simulink model "reactionWheel"  (R2019b)
settings: Solver=VariableStepAuto  StartTime=0.0  StopTime=10.0  RelTol=1e-3
model workspace (MAT data in the model file):
  Omega_max = 0.5
libraries: simulink x3, aerolibutil x1
settings Model: Creator=brice  LastModifiedBy=brice

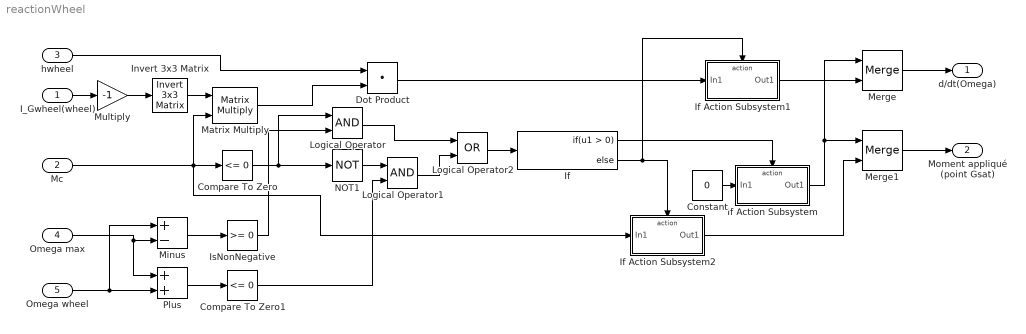
== system reactionWheel ==
  I_Gwheel(wheel) : Inport
  Mc : Inport  Port=2
  hwheel : Inport  Port=3
  Omega max : Inport  Port=4
  Omega wheel : Inport  Port=5
  Compare To Zero : simulink/Logic and Bit Operations/Compare To Zero  relop=<=  OutDataTypeStr=boolean
  Compare To Zero1 : simulink/Logic and Bit Operations/Compare To Zero  relop=<=  OutDataTypeStr=boolean
  Constant : Constant  Value=0
  Dot Product : DotProduct  InputSameDT=on  OutDataTypeStr=Inherit: Inherit via internal rule
  If : If
  If Action Subsystem : Subsystem  TreatAsAtomicUnit=on
  If Action Subsystem1 : Subsystem  TreatAsAtomicUnit=on
  If Action Subsystem2 : Subsystem  TreatAsAtomicUnit=on
  Invert 3x3 Matrix : aerolibutil/Invert  3x3 Matrix
  IsNonNegative : simulink/Logic and Bit Operations/Compare To Zero  relop=>=  OutDataTypeStr=boolean
  Logical Operator : Logic  AllPortsSameDT=off  OutDataTypeStr=boolean
  Logical Operator1 : Logic  AllPortsSameDT=off  OutDataTypeStr=boolean
  Logical Operator2 : Logic  Operator=OR  AllPortsSameDT=off  OutDataTypeStr=boolean
  Matrix Multiply : Product  Multiplication=Matrix(*)
  Merge : Merge
  Merge1 : Merge
  Minus : Sum  Inputs=+-
  Multiply : Gain  Gain=-1
  NOT1 : Logic  Operator=NOT  IconShape=distinctive  AllPortsSameDT=off  OutDataTypeStr=boolean
  Plus : Sum
  d/dt(Omega) : Outport
  Moment appliqué (point Gsat) : Outport  Port=2
  wires:
  Invert 3x3 Matrix/1 -> Matrix Multiply/1
  Mc/1 -> Matrix Multiply/2, Compare To Zero/1, If Action Subsystem2/1(In1)
  I_Gwheel(wheel)/1 -> Multiply/1
  Multiply/1 -> Invert 3x3 Matrix/1
  Compare To Zero/1 -> Logical Operator/1, NOT1/1
  Omega wheel/1 -> Minus/1, Plus/2
  Omega max/1 -> Plus/1, Minus/2
  Plus/1 -> Compare To Zero1/1
  Minus/1 -> IsNonNegative/1
  NOT1/1 -> Logical Operator1/1
  IsNonNegative/1 -> Logical Operator/2
  Compare To Zero1/1 -> Logical Operator1/2
  Logical Operator1/1 -> Logical Operator2/2
  Logical Operator/1 -> Logical Operator2/1
  Constant/1 -> If Action Subsystem/1(In1)
  Logical Operator2/1 -> If/1
  If/1 -> If Action Subsystem/Action
  If/2 -> If Action Subsystem2/Action, If Action Subsystem1/Action
  Dot Product/1 -> If Action Subsystem1/1(In1)
  If Action Subsystem/1(Out1) -> Merge1/1, Merge/1
  If Action Subsystem1/1(Out1) -> Merge/2
  Merge/1 -> d/dt(Omega)/1
  Merge1/1 -> Moment appliqué (point Gsat)/1
  If Action Subsystem2/1(Out1) -> Merge1/2
  Matrix Multiply/1 -> Dot Product/2
  hwheel/1 -> Dot Product/1

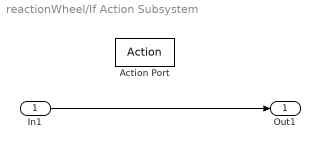
== system reactionWheel/If Action Subsystem ==
  In1 : Inport
  Action Port : ActionPort  ActionPortLabel=if(u1 > 0)
  Out1 : Outport
  wires:
  In1/1 -> Out1/1

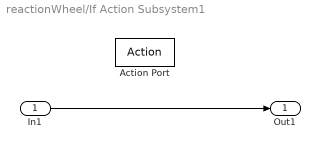
== system reactionWheel/If Action Subsystem1 ==
  In1 : Inport
  Action Port : ActionPort  ActionPortLabel=else
  Out1 : Outport
  wires:
  In1/1 -> Out1/1

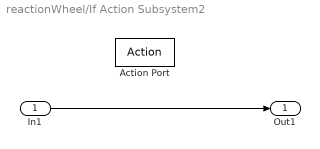
== system reactionWheel/If Action Subsystem2 ==
  In1 : Inport
  Action Port : ActionPort  ActionPortLabel=else
  Out1 : Outport
  wires:
  In1/1 -> Out1/1
